simulink model "EPA_Jumper"  (R2018a)
settings: Solver=FixedStepDiscrete  StartTime=0.0  StopTime=inf  FixedStep=0.001  RelTol=1e-3  EnableMultiTasking=on
model workspace (MAT data in the model file):
  MCOS : class17 (value not decoded)
values from neighbouring files (symbols this model uses):
  bits_current = 12    [Init_EPA_Jumper.m]
  bits_Kd = 12    [Init_EPA_Jumper.m]
  bits_Kp = 12    [Init_EPA_Jumper.m]
  bits_position = 16    [Init_EPA_Jumper.m]
  bits_velocity = 12    [Init_EPA_Jumper.m]
  KD_MAX = 5.0    (= 5)    [Init_EPA_Jumper.m]
  KD_MIN = 0.0    (= 0)    [Init_EPA_Jumper.m]
  KP_MAX = 500.0    (= 500)    [Init_EPA_Jumper.m]
  KP_MIN = 0.0    (= 0)    [Init_EPA_Jumper.m]
  P_MAX = 95.5    [Init_EPA_Jumper.m]
  P_MIN = -95.5    [Init_EPA_Jumper.m]
  PressureFilter_CutOffFreq = 20    [Init_EPA_Jumper.m]
  PressureFilter_Gain = 1    [Init_EPA_Jumper.m]
  ReadingVoltage = 5    [Init_EPA_Jumper.m]
  T_MAX = 18.0    (= 18)    [Init_EPA_Jumper.m]
  T_MIN = -18.0    (= -18)    [Init_EPA_Jumper.m]
  V_MAX = 45.0    (= 45)    [Init_EPA_Jumper.m]
  V_MIN = -45.0    (= -45)    [Init_EPA_Jumper.m]
  voltageBias = -2.5    [Init_EPA_Jumper.m]
  voltageMultiplier = 2.5    [Init_EPA_Jumper.m]
  VoltageResolution = 1023.0    (= 1023)    [Init_EPA_Jumper.m]
libraries: xpcethercatlib x76, slrtlib x15, simulink x10, peGeneralControl x9
(part 2 of 3)

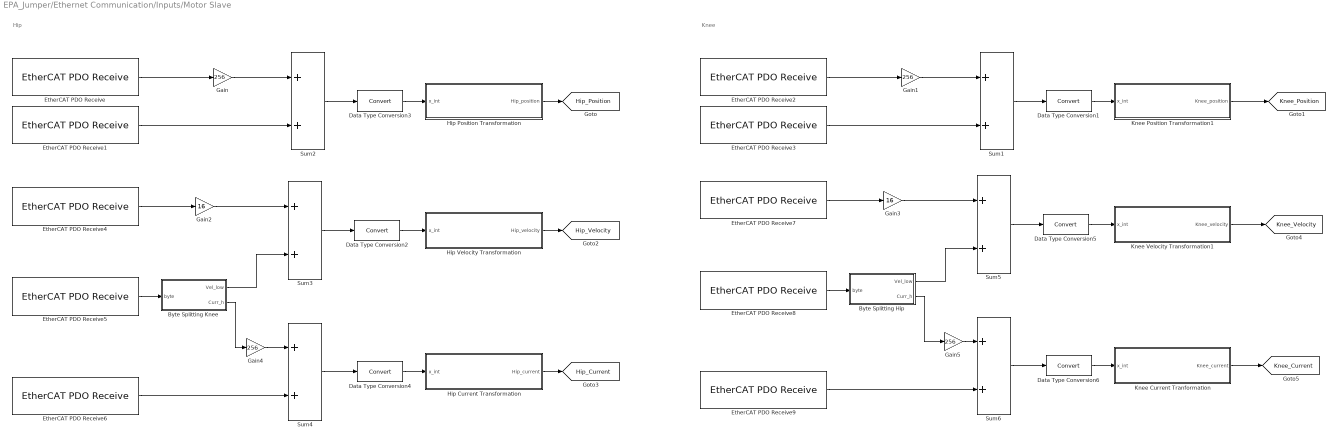
== system EPA_Jumper/Ethernet Communication/Inputs/Motor Slave ==
  note: Hip
  note: Knee
  Byte Splitting Hip : MATLAB Function  TreatAsAtomicUnit=on
  Byte Splitting Knee : MATLAB Function  TreatAsAtomicUnit=on
  Data Type Conversion{1..6} (6 alike) : DataTypeConversion
  EtherCAT PDO Receive : xpcethercatlib/EtherCAT PDO Receive  Priority=2  sig_name=Motors.Inputs.Byte0  sig_offset=464  sig_type=uint8  type_size=8  sig_dim=1  device_id=0  sample_time=0.001000
      settings: SourceProductName=Simulink Real-Time  SourceProductBaseCode=XP
  EtherCAT PDO Receive1 : xpcethercatlib/EtherCAT PDO Receive  Priority=2  sig_name=Motors.Inputs.Byte1  sig_offset=472  sig_type=uint8  type_size=8  sig_dim=1  device_id=0  sample_time=0.001000
      settings: SourceProductName=Simulink Real-Time  SourceProductBaseCode=XP
  EtherCAT PDO Receive2 : xpcethercatlib/EtherCAT PDO Receive  Priority=2  sig_name=Motors.Inputs.Byte5  sig_offset=504  sig_type=uint8  type_size=8  sig_dim=1  device_id=0  sample_time=0.001000
      settings: SourceProductName=Simulink Real-Time  SourceProductBaseCode=XP
  EtherCAT PDO Receive3 : xpcethercatlib/EtherCAT PDO Receive  Priority=2  sig_name=Motors.Inputs.Byte6  sig_offset=512  sig_type=uint8  type_size=8  sig_dim=1  device_id=0  sample_time=0.001000
      settings: SourceProductName=Simulink Real-Time  SourceProductBaseCode=XP
  EtherCAT PDO Receive4 : xpcethercatlib/EtherCAT PDO Receive  Priority=2  sig_name=Motors.Inputs.Byte2  sig_offset=480  sig_type=uint8  type_size=8  sig_dim=1  device_id=0  sample_time=0.001000
      settings: SourceProductName=Simulink Real-Time  SourceProductBaseCode=XP
  EtherCAT PDO Receive5 : xpcethercatlib/EtherCAT PDO Receive  Priority=2  sig_name=Motors.Inputs.Byte3  sig_offset=488  sig_type=uint8  type_size=8  sig_dim=1  device_id=0  sample_time=0.001000
      settings: SourceProductName=Simulink Real-Time  SourceProductBaseCode=XP
  EtherCAT PDO Receive6 : xpcethercatlib/EtherCAT PDO Receive  Priority=2  sig_name=Motors.Inputs.Byte4  sig_offset=496  sig_type=uint8  type_size=8  sig_dim=1  device_id=0  sample_time=0.001000
      settings: SourceProductName=Simulink Real-Time  SourceProductBaseCode=XP
  EtherCAT PDO Receive7 : xpcethercatlib/EtherCAT PDO Receive  Priority=2  sig_name=Motors.Inputs.Byte7  sig_offset=520  sig_type=uint8  type_size=8  sig_dim=1  device_id=0  sample_time=0.001000
      settings: SourceProductName=Simulink Real-Time  SourceProductBaseCode=XP
  EtherCAT PDO Receive8 : xpcethercatlib/EtherCAT PDO Receive  Priority=2  sig_name=Motors.Inputs.Byte8  sig_offset=528  sig_type=uint8  type_size=8  sig_dim=1  device_id=0  sample_time=0.001000
      settings: SourceProductName=Simulink Real-Time  SourceProductBaseCode=XP
  EtherCAT PDO Receive9 : xpcethercatlib/EtherCAT PDO Receive  Priority=2  sig_name=Motors.Inputs.Byte9  sig_offset=536  sig_type=uint8  type_size=8  sig_dim=1  device_id=0  sample_time=0.001000
      settings: SourceProductName=Simulink Real-Time  SourceProductBaseCode=XP
  Gain{,1,4..5} (4 alike) : Gain  Gain=256
  Gain2 : Gain  Gain=16
  Gain3 : Gain  Gain=16
  Hip Current Transformation : MATLAB Function  TreatAsAtomicUnit=on
  Hip Position Transformation : MATLAB Function  TreatAsAtomicUnit=on
  Hip Velocity Transformation : MATLAB Function  TreatAsAtomicUnit=on
  Knee Current Tranformation : MATLAB Function  TreatAsAtomicUnit=on
  Knee Position Transformation1 : MATLAB Function  TreatAsAtomicUnit=on
  Knee Velocity Transformation1 : MATLAB Function  TreatAsAtomicUnit=on
  Sum{1..6} (6 alike) : Sum
  tag scope: Hip_Current=global, Hip_Position=global, Hip_Velocity=global, Knee_Current=global, Knee_Position=global, Knee_Velocity=global
  wires:
  EtherCAT PDO Receive/1 -> Gain/1
  Sum2/1 -> Data Type Conversion3/1
  Data Type Conversion3/1 -> Hip Position Transformation/1(x_int)
  Gain/1 -> Sum2/1
  EtherCAT PDO Receive1/1 -> Sum2/2
  EtherCAT PDO Receive3/1 -> Sum1/2
  Gain1/1 -> Sum1/1
  Data Type Conversion1/1 -> Knee Position Transformation1/1(x_int)
  EtherCAT PDO Receive2/1 -> Gain1/1
  Sum1/1 -> Data Type Conversion1/1
  EtherCAT PDO Receive5/1 -> Byte Splitting Knee/1(byte)
  EtherCAT PDO Receive4/1 -> Gain2/1
  Gain2/1 -> Sum3/1
  Byte Splitting Knee/1(Vel_low) -> Sum3/2
  EtherCAT PDO Receive6/1 -> Sum4/2
  Data Type Conversion2/1 -> Hip Velocity Transformation/1(x_int)
  Sum3/1 -> Data Type Conversion2/1
  Data Type Conversion4/1 -> Hip Current Transformation/1(x_int)
  Sum4/1 -> Data Type Conversion4/1
  EtherCAT PDO Receive7/1 -> Gain3/1
  Sum5/1 -> Data Type Conversion5/1
  Gain3/1 -> Sum5/1
  EtherCAT PDO Receive9/1 -> Sum6/2
  EtherCAT PDO Receive8/1 -> Byte Splitting Hip/1(byte)
  Byte Splitting Hip/2(Curr_h) -> Gain5/1
  Sum6/1 -> Data Type Conversion6/1
  Byte Splitting Hip/1(Vel_low) -> Sum5/2
  Hip Position Transformation/1(Hip_position) -> [Hip_Position]
  Hip Velocity Transformation/1(Hip_velocity) -> [Hip_Velocity]
  Hip Current Transformation/1(Hip_current) -> [Hip_Current]
  Knee Position Transformation1/1(Knee_position) -> [Knee_Position]
  Knee Velocity Transformation1/1(Knee_velocity) -> [Knee_Velocity]
  Data Type Conversion5/1 -> Knee Velocity Transformation1/1(x_int)
  Knee Current Tranformation/1(Knee_current) -> [Knee_Current]
  Data Type Conversion6/1 -> Knee Current Tranformation/1(x_int)
  Gain4/1 -> Sum4/1
  Byte Splitting Knee/2(Curr_h) -> Gain4/1
  Gain5/1 -> Sum6/1

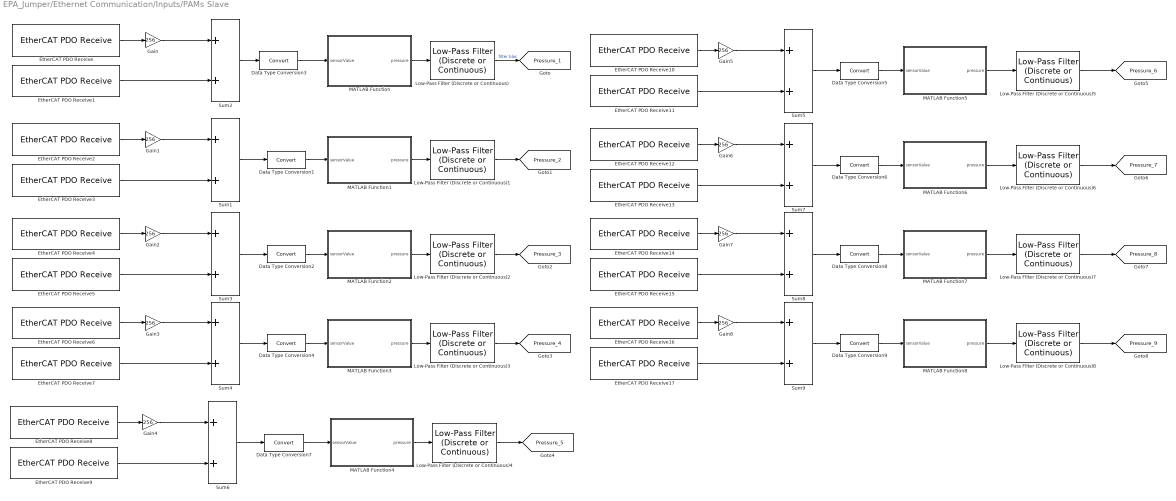
== system EPA_Jumper/Ethernet Communication/Inputs/PAMs Slave ==
  Data Type Conversion{1..9} (9 alike) : DataTypeConversion
  EtherCAT PDO Receive : xpcethercatlib/EtherCAT PDO Receive  Priority=2  sig_name=PAMs.Inputs.Byte0  sig_offset=720  sig_type=uint8  type_size=8  sig_dim=1  device_id=0  sample_time=0.001000
      settings: SourceProductName=Simulink Real-Time  SourceProductBaseCode=XP
  EtherCAT PDO Receive1 : xpcethercatlib/EtherCAT PDO Receive  Priority=2  sig_name=PAMs.Inputs.Byte1  sig_offset=728  sig_type=uint8  type_size=8  sig_dim=1  device_id=0  sample_time=0.001000
      settings: SourceProductName=Simulink Real-Time  SourceProductBaseCode=XP
  EtherCAT PDO Receive10 : xpcethercatlib/EtherCAT PDO Receive  Priority=2  sig_name=PAMs.Inputs.Byte10  sig_offset=800  sig_type=uint8  type_size=8  sig_dim=1  device_id=0  sample_time=0.001000
      settings: SourceProductName=Simulink Real-Time  SourceProductBaseCode=XP
  EtherCAT PDO Receive11 : xpcethercatlib/EtherCAT PDO Receive  Priority=2  sig_name=PAMs.Inputs.Byte11  sig_offset=808  sig_type=uint8  type_size=8  sig_dim=1  device_id=0  sample_time=0.001000
      settings: SourceProductName=Simulink Real-Time  SourceProductBaseCode=XP
  EtherCAT PDO Receive12 : xpcethercatlib/EtherCAT PDO Receive  Priority=2  sig_name=PAMs.Inputs.Byte12  sig_offset=816  sig_type=uint8  type_size=8  sig_dim=1  device_id=0  sample_time=0.001000
      settings: SourceProductName=Simulink Real-Time  SourceProductBaseCode=XP
  EtherCAT PDO Receive13 : xpcethercatlib/EtherCAT PDO Receive  Priority=2  sig_name=PAMs.Inputs.Byte13  sig_offset=824  sig_type=uint8  type_size=8  sig_dim=1  device_id=0  sample_time=0.001000
      settings: SourceProductName=Simulink Real-Time  SourceProductBaseCode=XP
  EtherCAT PDO Receive14 : xpcethercatlib/EtherCAT PDO Receive  Priority=2  sig_name=PAMs.Inputs.Byte14  sig_offset=832  sig_type=uint8  type_size=8  sig_dim=1  device_id=0  sample_time=0.001000
      settings: SourceProductName=Simulink Real-Time  SourceProductBaseCode=XP
  EtherCAT PDO Receive15 : xpcethercatlib/EtherCAT PDO Receive  Priority=2  sig_name=PAMs.Inputs.Byte15  sig_offset=840  sig_type=uint8  type_size=8  sig_dim=1  device_id=0  sample_time=0.001000
      settings: SourceProductName=Simulink Real-Time  SourceProductBaseCode=XP
  EtherCAT PDO Receive16 : xpcethercatlib/EtherCAT PDO Receive  Priority=2  sig_name=PAMs.Inputs.Byte16  sig_offset=848  sig_type=uint8  type_size=8  sig_dim=1  device_id=0  sample_time=0.001000
      settings: SourceProductName=Simulink Real-Time  SourceProductBaseCode=XP
  EtherCAT PDO Receive17 : xpcethercatlib/EtherCAT PDO Receive  Priority=2  sig_name=PAMs.Inputs.Byte17  sig_offset=856  sig_type=uint8  type_size=8  sig_dim=1  device_id=0  sample_time=0.001000
      settings: SourceProductName=Simulink Real-Time  SourceProductBaseCode=XP
  EtherCAT PDO Receive2 : xpcethercatlib/EtherCAT PDO Receive  Priority=2  sig_name=PAMs.Inputs.Byte2  sig_offset=736  sig_type=uint8  type_size=8  sig_dim=1  device_id=0  sample_time=0.001000
      settings: SourceProductName=Simulink Real-Time  SourceProductBaseCode=XP
  EtherCAT PDO Receive3 : xpcethercatlib/EtherCAT PDO Receive  Priority=2  sig_name=PAMs.Inputs.Byte3  sig_offset=744  sig_type=uint8  type_size=8  sig_dim=1  device_id=0  sample_time=0.001000
      settings: SourceProductName=Simulink Real-Time  SourceProductBaseCode=XP
  EtherCAT PDO Receive4 : xpcethercatlib/EtherCAT PDO Receive  Priority=2  sig_name=PAMs.Inputs.Byte4  sig_offset=752  sig_type=uint8  type_size=8  sig_dim=1  device_id=0  sample_time=0.001000
      settings: SourceProductName=Simulink Real-Time  SourceProductBaseCode=XP
  EtherCAT PDO Receive5 : xpcethercatlib/EtherCAT PDO Receive  Priority=2  sig_name=PAMs.Inputs.Byte5  sig_offset=760  sig_type=uint8  type_size=8  sig_dim=1  device_id=0  sample_time=0.001000
      settings: SourceProductName=Simulink Real-Time  SourceProductBaseCode=XP
  EtherCAT PDO Receive6 : xpcethercatlib/EtherCAT PDO Receive  Priority=2  sig_name=PAMs.Inputs.Byte6  sig_offset=768  sig_type=uint8  type_size=8  sig_dim=1  device_id=0  sample_time=0.001000
      settings: SourceProductName=Simulink Real-Time  SourceProductBaseCode=XP
  EtherCAT PDO Receive7 : xpcethercatlib/EtherCAT PDO Receive  Priority=2  sig_name=PAMs.Inputs.Byte7  sig_offset=776  sig_type=uint8  type_size=8  sig_dim=1  device_id=0  sample_time=0.001000
      settings: SourceProductName=Simulink Real-Time  SourceProductBaseCode=XP
  EtherCAT PDO Receive8 : xpcethercatlib/EtherCAT PDO Receive  Priority=2  sig_name=PAMs.Inputs.Byte8  sig_offset=784  sig_type=uint8  type_size=8  sig_dim=1  device_id=0  sample_time=0.001000
      settings: SourceProductName=Simulink Real-Time  SourceProductBaseCode=XP
  EtherCAT PDO Receive9 : xpcethercatlib/EtherCAT PDO Receive  Priority=2  sig_name=PAMs.Inputs.Byte9  sig_offset=792  sig_type=uint8  type_size=8  sig_dim=1  device_id=0  sample_time=0.001000
      settings: SourceProductName=Simulink Real-Time  SourceProductBaseCode=XP
  Gain{,1..8} (9 alike) : Gain  Gain=256
  Low-Pass Filter (Discrete or Continuous){,1..8} (9 alike) : peGeneralControl/Low-Pass Filter (Discrete or Continuous)  K=PressureFilter_Gain  T=1/PressureFilter_CutOffFreq  B=inf  A=-inf  Ts=-1
  MATLAB Function : MATLAB Function  TreatAsAtomicUnit=on
  MATLAB Function1 : MATLAB Function  TreatAsAtomicUnit=on
  MATLAB Function2 : MATLAB Function  TreatAsAtomicUnit=on
  MATLAB Function3 : MATLAB Function  TreatAsAtomicUnit=on
  MATLAB Function4 : MATLAB Function  TreatAsAtomicUnit=on
  MATLAB Function5 : MATLAB Function  TreatAsAtomicUnit=on
  MATLAB Function6 : MATLAB Function  TreatAsAtomicUnit=on
  MATLAB Function7 : MATLAB Function  TreatAsAtomicUnit=on
  MATLAB Function8 : MATLAB Function  TreatAsAtomicUnit=on
  Sum{1..9} (9 alike) : Sum
  tag scope: Pressure_1=global, Pressure_2=global, Pressure_3=global, Pressure_4=global, Pressure_5=global, Pressure_6=global, Pressure_7=global, Pressure_8=global, Pressure_9=global
  wires:
  EtherCAT PDO Receive1/1 -> Sum2/2
  Sum2/1 -> Data Type Conversion3/1
  EtherCAT PDO Receive/1 -> Gain/1
  Gain/1 -> Sum2/1
  Data Type Conversion3/1 -> MATLAB Function/1(sensorValue)
  Gain1/1 -> Sum1/1
  EtherCAT PDO Receive3/1 -> Sum1/2
  EtherCAT PDO Receive2/1 -> Gain1/1
  Data Type Conversion1/1 -> MATLAB Function1/1(sensorValue)
  Sum1/1 -> Data Type Conversion1/1
  Data Type Conversion2/1 -> MATLAB Function2/1(sensorValue)
  EtherCAT PDO Receive4/1 -> Gain2/1
  Gain2/1 -> Sum3/1
  Sum3/1 -> Data Type Conversion2/1
  EtherCAT PDO Receive5/1 -> Sum3/2
  Sum4/1 -> Data Type Conversion4/1
  Data Type Conversion4/1 -> MATLAB Function3/1(sensorValue)
  EtherCAT PDO Receive6/1 -> Gain3/1
  Gain3/1 -> Sum4/1
  EtherCAT PDO Receive7/1 -> Sum4/2
  Gain4/1 -> Sum6/1
  Sum6/1 -> Data Type Conversion7/1
  EtherCAT PDO Receive8/1 -> Gain4/1
  Data Type Conversion5/1 -> MATLAB Function5/1(sensorValue)
  EtherCAT PDO Receive10/1 -> Gain5/1
  Gain5/1 -> Sum5/1
  EtherCAT PDO Receive11/1 -> Sum5/2
  Data Type Conversion7/1 -> MATLAB Function4/1(sensorValue)
  EtherCAT PDO Receive15/1 -> Sum8/2
  Gain7/1 -> Sum8/1
  EtherCAT PDO Receive14/1 -> Gain7/1
  Data Type Conversion8/1 -> MATLAB Function7/1(sensorValue)
  Sum7/1 -> Data Type Conversion6/1
  Data Type Conversion6/1 -> MATLAB Function6/1(sensorValue)
  EtherCAT PDO Receive12/1 -> Gain6/1
  Sum5/1 -> Data Type Conversion5/1
  Sum8/1 -> Data Type Conversion8/1
  EtherCAT PDO Receive9/1 -> Sum6/2
  Gain6/1 -> Sum7/1
  EtherCAT PDO Receive13/1 -> Sum7/2
  MATLAB Function/1(pressure) -> Low-Pass Filter (Discrete or Continuous)/1
  MATLAB Function1/1(pressure) -> Low-Pass Filter (Discrete or Continuous)1/1
  MATLAB Function2/1(pressure) -> Low-Pass Filter (Discrete or Continuous)2/1
  MATLAB Function3/1(pressure) -> Low-Pass Filter (Discrete or Continuous)3/1
  MATLAB Function4/1(pressure) -> Low-Pass Filter (Discrete or Continuous)4/1
  MATLAB Function5/1(pressure) -> Low-Pass Filter (Discrete or Continuous)5/1
  MATLAB Function6/1(pressure) -> Low-Pass Filter (Discrete or Continuous)6/1
  MATLAB Function7/1(pressure) -> Low-Pass Filter (Discrete or Continuous)7/1
  Sum9/1 -> Data Type Conversion9/1
  EtherCAT PDO Receive16/1 -> Gain8/1
  Data Type Conversion9/1 -> MATLAB Function8/1(sensorValue)
  Gain8/1 -> Sum9/1
  MATLAB Function8/1(pressure) -> Low-Pass Filter (Discrete or Continuous)8/1
  EtherCAT PDO Receive17/1 -> Sum9/2
  Low-Pass Filter (Discrete or Continuous)/1 -> [Pressure_1]  "filter bloc"
  Low-Pass Filter (Discrete or Continuous)1/1 -> [Pressure_2]
  Low-Pass Filter (Discrete or Continuous)2/1 -> [Pressure_3]
  Low-Pass Filter (Discrete or Continuous)3/1 -> [Pressure_4]
  Low-Pass Filter (Discrete or Continuous)4/1 -> [Pressure_5]
  Low-Pass Filter (Discrete or Continuous)5/1 -> [Pressure_6]
  Low-Pass Filter (Discrete or Continuous)6/1 -> [Pressure_7]
  Low-Pass Filter (Discrete or Continuous)7/1 -> [Pressure_8]
  Low-Pass Filter (Discrete or Continuous)8/1 -> [Pressure_9]

== system EPA_Jumper/Ethernet Communication/Outputs/GRF Slave ==
  Data Type Conversion13 : DataTypeConversion
  EtherCAT PDO Transmit 2 : xpcethercatlib/EtherCAT PDO Transmit   Priority=3  sig_name=GRF.Outputs.Byte0  sig_offset=208  sig_type=uint8  type_size=8  sig_dim=1  device_id=0  sample_time=0.001000
      settings: SourceProductName=Simulink Real-Time  SourceProductBaseCode=XP
  wires:
  Data Type Conversion13/1 -> EtherCAT PDO Transmit 2/1
  [GRF_Operation_Mode] -> Data Type Conversion13/1

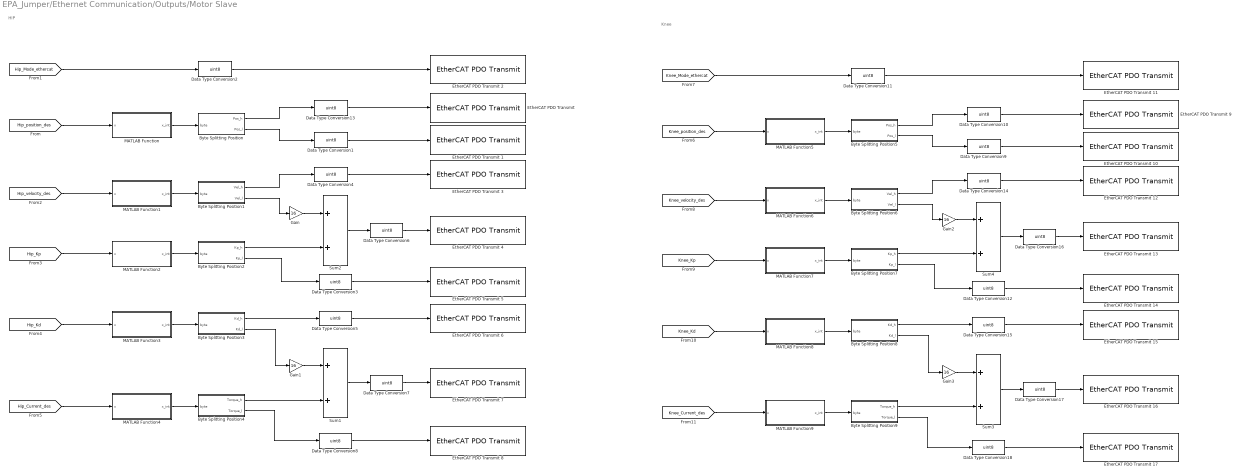
== system EPA_Jumper/Ethernet Communication/Outputs/Motor Slave ==
  note: HIP
  note: Knee
  Byte Splitting Position : MATLAB Function  TreatAsAtomicUnit=on
  Byte Splitting Position1 : MATLAB Function  TreatAsAtomicUnit=on
  Byte Splitting Position2 : MATLAB Function  TreatAsAtomicUnit=on
  Byte Splitting Position3 : MATLAB Function  TreatAsAtomicUnit=on
  Byte Splitting Position4 : MATLAB Function  TreatAsAtomicUnit=on
  Byte Splitting Position5 : MATLAB Function  TreatAsAtomicUnit=on
  Byte Splitting Position6 : MATLAB Function  TreatAsAtomicUnit=on
  Byte Splitting Position7 : MATLAB Function  TreatAsAtomicUnit=on
  Byte Splitting Position8 : MATLAB Function  TreatAsAtomicUnit=on
  Byte Splitting Position9 : MATLAB Function  TreatAsAtomicUnit=on
  Data Type Conversion{1,3..18} (17 alike) : DataTypeConversion  OutDataTypeStr=uint8
  Data Type Conversion2 : DataTypeConversion  OutDataTypeStr=uint8  RndMeth=Ceiling
  "EtherCAT PDO Transmit " : xpcethercatlib/EtherCAT PDO Transmit   Priority=3  sig_name=Motors.Outputs.Byte1  sig_offset=472  sig_type=uint8  type_size=8  sig_dim=1  device_id=0  sample_time=0.001000
      settings: SourceProductName=Simulink Real-Time  SourceProductBaseCode=XP
  EtherCAT PDO Transmit 1 : xpcethercatlib/EtherCAT PDO Transmit   Priority=3  sig_name=Motors.Outputs.Byte2  sig_offset=480  sig_type=uint8  type_size=8  sig_dim=1  device_id=0  sample_time=0.001000
      settings: SourceProductName=Simulink Real-Time  SourceProductBaseCode=XP
  EtherCAT PDO Transmit 10 : xpcethercatlib/EtherCAT PDO Transmit   Priority=3  sig_name=Motors.Outputs.Byte11  sig_offset=552  sig_type=uint8  type_size=8  sig_dim=1  device_id=0  sample_time=0.001000
      settings: SourceProductName=Simulink Real-Time  SourceProductBaseCode=XP
  EtherCAT PDO Transmit 11 : xpcethercatlib/EtherCAT PDO Transmit   Priority=3  sig_name=Motors.Outputs.Byte9  sig_offset=536  sig_type=uint8  type_size=8  sig_dim=1  device_id=0  sample_time=0.001000
      settings: SourceProductName=Simulink Real-Time  SourceProductBaseCode=XP
  EtherCAT PDO Transmit 12 : xpcethercatlib/EtherCAT PDO Transmit   Priority=3  sig_name=Motors.Outputs.Byte12  sig_offset=560  sig_type=uint8  type_size=8  sig_dim=1  device_id=0  sample_time=0.001000
      settings: SourceProductName=Simulink Real-Time  SourceProductBaseCode=XP
  EtherCAT PDO Transmit 13 : xpcethercatlib/EtherCAT PDO Transmit   Priority=3  sig_name=Motors.Outputs.Byte13  sig_offset=568  sig_type=uint8  type_size=8  sig_dim=1  device_id=0  sample_time=0.001000
      settings: SourceProductName=Simulink Real-Time  SourceProductBaseCode=XP
  EtherCAT PDO Transmit 14 : xpcethercatlib/EtherCAT PDO Transmit   Priority=3  sig_name=Motors.Outputs.Byte14  sig_offset=576  sig_type=uint8  type_size=8  sig_dim=1  device_id=0  sample_time=0.001000
      settings: SourceProductName=Simulink Real-Time  SourceProductBaseCode=XP
  EtherCAT PDO Transmit 15 : xpcethercatlib/EtherCAT PDO Transmit   Priority=3  sig_name=Motors.Outputs.Byte15  sig_offset=584  sig_type=uint8  type_size=8  sig_dim=1  device_id=0  sample_time=0.001000
      settings: SourceProductName=Simulink Real-Time  SourceProductBaseCode=XP
  EtherCAT PDO Transmit 16 : xpcethercatlib/EtherCAT PDO Transmit   Priority=3  sig_name=Motors.Outputs.Byte16  sig_offset=592  sig_type=uint8  type_size=8  sig_dim=1  device_id=0  sample_time=0.001000
      settings: SourceProductName=Simulink Real-Time  SourceProductBaseCode=XP
  EtherCAT PDO Transmit 17 : xpcethercatlib/EtherCAT PDO Transmit   Priority=3  sig_name=Motors.Outputs.Byte17  sig_offset=600  sig_type=uint8  type_size=8  sig_dim=1  device_id=0  sample_time=0.001000
      settings: SourceProductName=Simulink Real-Time  SourceProductBaseCode=XP
  EtherCAT PDO Transmit 2 : xpcethercatlib/EtherCAT PDO Transmit   Priority=3  sig_name=Motors.Outputs.Byte0  sig_offset=464  sig_type=uint8  type_size=8  sig_dim=1  device_id=0  sample_time=0.001000
      settings: SourceProductName=Simulink Real-Time  SourceProductBaseCode=XP
  EtherCAT PDO Transmit 3 : xpcethercatlib/EtherCAT PDO Transmit   Priority=3  sig_name=Motors.Outputs.Byte3  sig_offset=488  sig_type=uint8  type_size=8  sig_dim=1  device_id=0  sample_time=0.001000
      settings: SourceProductName=Simulink Real-Time  SourceProductBaseCode=XP
  EtherCAT PDO Transmit 4 : xpcethercatlib/EtherCAT PDO Transmit   Priority=3  sig_name=Motors.Outputs.Byte4  sig_offset=496  sig_type=uint8  type_size=8  sig_dim=1  device_id=0  sample_time=0.001000
      settings: SourceProductName=Simulink Real-Time  SourceProductBaseCode=XP
  EtherCAT PDO Transmit 5 : xpcethercatlib/EtherCAT PDO Transmit   Priority=3  sig_name=Motors.Outputs.Byte5  sig_offset=504  sig_type=uint8  type_size=8  sig_dim=1  device_id=0  sample_time=0.001000
      settings: SourceProductName=Simulink Real-Time  SourceProductBaseCode=XP
  EtherCAT PDO Transmit 6 : xpcethercatlib/EtherCAT PDO Transmit   Priority=3  sig_name=Motors.Outputs.Byte6  sig_offset=512  sig_type=uint8  type_size=8  sig_dim=1  device_id=0  sample_time=0.001000
      settings: SourceProductName=Simulink Real-Time  SourceProductBaseCode=XP
  EtherCAT PDO Transmit 7 : xpcethercatlib/EtherCAT PDO Transmit   Priority=3  sig_name=Motors.Outputs.Byte7  sig_offset=520  sig_type=uint8  type_size=8  sig_dim=1  device_id=0  sample_time=0.001000
      settings: SourceProductName=Simulink Real-Time  SourceProductBaseCode=XP
  EtherCAT PDO Transmit 8 : xpcethercatlib/EtherCAT PDO Transmit   Priority=3  sig_name=Motors.Outputs.Byte8  sig_offset=528  sig_type=uint8  type_size=8  sig_dim=1  device_id=0  sample_time=0.001000
      settings: SourceProductName=Simulink Real-Time  SourceProductBaseCode=XP
  EtherCAT PDO Transmit 9 : xpcethercatlib/EtherCAT PDO Transmit   Priority=3  sig_name=Motors.Outputs.Byte10  sig_offset=544  sig_type=uint8  type_size=8  sig_dim=1  device_id=0  sample_time=0.001000
      settings: SourceProductName=Simulink Real-Time  SourceProductBaseCode=XP
  Gain{,1..3} (4 alike) : Gain  Gain=16
  MATLAB Function : MATLAB Function  TreatAsAtomicUnit=on
  MATLAB Function1 : MATLAB Function  TreatAsAtomicUnit=on
  MATLAB Function2 : MATLAB Function  TreatAsAtomicUnit=on
  MATLAB Function3 : MATLAB Function  TreatAsAtomicUnit=on
  MATLAB Function4 : MATLAB Function  TreatAsAtomicUnit=on
  MATLAB Function5 : MATLAB Function  TreatAsAtomicUnit=on
  MATLAB Function6 : MATLAB Function  TreatAsAtomicUnit=on
  MATLAB Function7 : MATLAB Function  TreatAsAtomicUnit=on
  MATLAB Function8 : MATLAB Function  TreatAsAtomicUnit=on
  MATLAB Function9 : MATLAB Function  TreatAsAtomicUnit=on
  Sum{1..4} (4 alike) : Sum
  wires:
  [Hip_position_des] -> MATLAB Function/1(x)
  MATLAB Function/1(x_int) -> Byte Splitting Position/1(byte)
  Byte Splitting Position/1(Pos_h) -> Data Type Conversion13/1
  Byte Splitting Position/2(Pos_l) -> Data Type Conversion1/1
  Data Type Conversion13/1 -> "EtherCAT PDO Transmit "/1
  Data Type Conversion1/1 -> EtherCAT PDO Transmit 1/1
  [Hip_Mode_ethercat] -> Data Type Conversion2/1
  Data Type Conversion2/1 -> EtherCAT PDO Transmit 2/1
  MATLAB Function1/1(x_int) -> Byte Splitting Position1/1(byte)
  Byte Splitting Position1/1(Vel_h) -> Data Type Conversion4/1
  Byte Splitting Position1/2(Vel_l) -> Gain/1
  [Hip_velocity_des] -> MATLAB Function1/1(x)
  Data Type Conversion4/1 -> EtherCAT PDO Transmit 3/1
  Gain/1 -> Sum2/1
  Sum2/1 -> Data Type Conversion6/1
  [Hip_Kp] -> MATLAB Function2/1(x)
  MATLAB Function2/1(x_int) -> Byte Splitting Position2/1(byte)
  Byte Splitting Position2/1(Kp_h) -> Sum2/2
  Data Type Conversion3/1 -> EtherCAT PDO Transmit 5/1
  Byte Splitting Position2/2(Kp_l) -> Data Type Conversion3/1
  [Hip_Kd] -> MATLAB Function3/1(x)
  MATLAB Function3/1(x_int) -> Byte Splitting Position3/1(byte)
  Byte Splitting Position3/2(Kd_l) -> Gain1/1
  Byte Splitting Position3/1(Kd_h) -> Data Type Conversion5/1
  Sum1/1 -> Data Type Conversion7/1
  Data Type Conversion5/1 -> EtherCAT PDO Transmit 6/1
  Gain1/1 -> Sum1/1
  Data Type Conversion6/1 -> EtherCAT PDO Transmit 4/1
  Data Type Conversion7/1 -> EtherCAT PDO Transmit 7/1
  [Hip_Current_des] -> MATLAB Function4/1(x)
  MATLAB Function4/1(x_int) -> Byte Splitting Position4/1(byte)
  Byte Splitting Position4/2(Torque_l) -> Data Type Conversion8/1
  Byte Splitting Position4/1(Torque_h) -> Sum1/2
  Data Type Conversion8/1 -> EtherCAT PDO Transmit 8/1
  Byte Splitting Position9/2(Torque_l) -> Data Type Conversion18/1
  Data Type Conversion15/1 -> EtherCAT PDO Transmit 15/1
  Byte Splitting Position8/2(Kd_l) -> Gain3/1
  Data Type Conversion17/1 -> EtherCAT PDO Transmit 16/1
  MATLAB Function5/1(x_int) -> Byte Splitting Position5/1(byte)
  Data Type Conversion10/1 -> EtherCAT PDO Transmit 9/1
  Data Type Conversion18/1 -> EtherCAT PDO Transmit 17/1
  MATLAB Function9/1(x_int) -> Byte Splitting Position9/1(byte)
  Byte Splitting Position9/1(Torque_h) -> Sum3/2
  [Knee_Mode_ethercat] -> Data Type Conversion11/1
  Data Type Conversion14/1 -> EtherCAT PDO Transmit 12/1
  [Knee_Kp] -> MATLAB Function7/1(x)
  MATLAB Function7/1(x_int) -> Byte Splitting Position7/1(byte)
  Byte Splitting Position7/2(Kp_l) -> Data Type Conversion12/1
  Byte Splitting Position8/1(Kd_h) -> Data Type Conversion15/1
  [Knee_Current_des] -> MATLAB Function9/1(x)
  Byte Splitting Position6/2(Vel_l) -> Gain2/1
  Data Type Conversion12/1 -> EtherCAT PDO Transmit 14/1
  Sum3/1 -> Data Type Conversion17/1
  Byte Splitting Position7/1(Kp_h) -> Sum4/2
  Byte Splitting Position5/2(Pos_l) -> Data Type Conversion9/1
  Data Type Conversion9/1 -> EtherCAT PDO Transmit 10/1
  Byte Splitting Position5/1(Pos_h) -> Data Type Conversion10/1
  Sum4/1 -> Data Type Conversion16/1
  Data Type Conversion11/1 -> EtherCAT PDO Transmit 11/1
  [Knee_velocity_des] -> MATLAB Function6/1(x)
  [Knee_position_des] -> MATLAB Function5/1(x)
  [Knee_Kd] -> MATLAB Function8/1(x)
  Gain2/1 -> Sum4/1
  Gain3/1 -> Sum3/1
  MATLAB Function8/1(x_int) -> Byte Splitting Position8/1(byte)
  Byte Splitting Position6/1(Vel_h) -> Data Type Conversion14/1
  MATLAB Function6/1(x_int) -> Byte Splitting Position6/1(byte)
  Data Type Conversion16/1 -> EtherCAT PDO Transmit 13/1

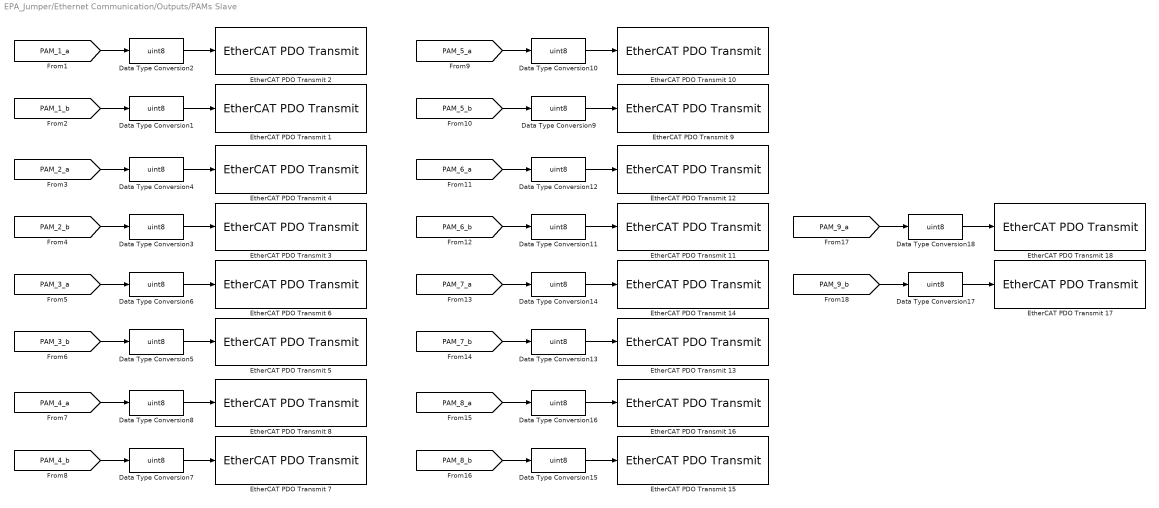
== system EPA_Jumper/Ethernet Communication/Outputs/PAMs Slave ==
  Data Type Conversion{1..18} (18 alike) : DataTypeConversion  OutDataTypeStr=uint8  RndMeth=Ceiling
  EtherCAT PDO Transmit 1 : xpcethercatlib/EtherCAT PDO Transmit   Priority=3  sig_name=PAMs.Outputs.Byte1  sig_offset=728  sig_type=uint8  type_size=8  sig_dim=1  device_id=0  sample_time=0.001000
      settings: SourceProductName=Simulink Real-Time  SourceProductBaseCode=XP
  EtherCAT PDO Transmit 10 : xpcethercatlib/EtherCAT PDO Transmit   Priority=3  sig_name=PAMs.Outputs.Byte8  sig_offset=784  sig_type=uint8  type_size=8  sig_dim=1  device_id=0  sample_time=0.001000
      settings: SourceProductName=Simulink Real-Time  SourceProductBaseCode=XP
  EtherCAT PDO Transmit 11 : xpcethercatlib/EtherCAT PDO Transmit   Priority=3  sig_name=PAMs.Outputs.Byte11  sig_offset=808  sig_type=uint8  type_size=8  sig_dim=1  device_id=0  sample_time=0.001000
      settings: SourceProductName=Simulink Real-Time  SourceProductBaseCode=XP
  EtherCAT PDO Transmit 12 : xpcethercatlib/EtherCAT PDO Transmit   Priority=3  sig_name=PAMs.Outputs.Byte10  sig_offset=800  sig_type=uint8  type_size=8  sig_dim=1  device_id=0  sample_time=0.001000
      settings: SourceProductName=Simulink Real-Time  SourceProductBaseCode=XP
  EtherCAT PDO Transmit 13 : xpcethercatlib/EtherCAT PDO Transmit   Priority=3  sig_name=PAMs.Outputs.Byte13  sig_offset=824  sig_type=uint8  type_size=8  sig_dim=1  device_id=0  sample_time=0.001000
      settings: SourceProductName=Simulink Real-Time  SourceProductBaseCode=XP
  EtherCAT PDO Transmit 14 : xpcethercatlib/EtherCAT PDO Transmit   Priority=3  sig_name=PAMs.Outputs.Byte12  sig_offset=816  sig_type=uint8  type_size=8  sig_dim=1  device_id=0  sample_time=0.001000
      settings: SourceProductName=Simulink Real-Time  SourceProductBaseCode=XP
  EtherCAT PDO Transmit 15 : xpcethercatlib/EtherCAT PDO Transmit   Priority=3  sig_name=PAMs.Outputs.Byte15  sig_offset=840  sig_type=uint8  type_size=8  sig_dim=1  device_id=0  sample_time=0.001000
      settings: SourceProductName=Simulink Real-Time  SourceProductBaseCode=XP
  EtherCAT PDO Transmit 16 : xpcethercatlib/EtherCAT PDO Transmit   Priority=3  sig_name=PAMs.Outputs.Byte14  sig_offset=832  sig_type=uint8  type_size=8  sig_dim=1  device_id=0  sample_time=0.001000
      settings: SourceProductName=Simulink Real-Time  SourceProductBaseCode=XP
  EtherCAT PDO Transmit 17 : xpcethercatlib/EtherCAT PDO Transmit   Priority=3  sig_name=PAMs.Outputs.Byte17  sig_offset=856  sig_type=uint8  type_size=8  sig_dim=1  device_id=0  sample_time=0.001000
      settings: SourceProductName=Simulink Real-Time  SourceProductBaseCode=XP
  EtherCAT PDO Transmit 18 : xpcethercatlib/EtherCAT PDO Transmit   Priority=3  sig_name=PAMs.Outputs.Byte16  sig_offset=848  sig_type=uint8  type_size=8  sig_dim=1  device_id=0  sample_time=0.001000
      settings: SourceProductName=Simulink Real-Time  SourceProductBaseCode=XP
  EtherCAT PDO Transmit 2 : xpcethercatlib/EtherCAT PDO Transmit   Priority=3  sig_name=PAMs.Outputs.Byte0  sig_offset=720  sig_type=uint8  type_size=8  sig_dim=1  device_id=0  sample_time=0.001000
      settings: SourceProductName=Simulink Real-Time  SourceProductBaseCode=XP
  EtherCAT PDO Transmit 3 : xpcethercatlib/EtherCAT PDO Transmit   Priority=3  sig_name=PAMs.Outputs.Byte3  sig_offset=744  sig_type=uint8  type_size=8  sig_dim=1  device_id=0  sample_time=0.001000
      settings: SourceProductName=Simulink Real-Time  SourceProductBaseCode=XP
  EtherCAT PDO Transmit 4 : xpcethercatlib/EtherCAT PDO Transmit   Priority=3  sig_name=PAMs.Outputs.Byte2  sig_offset=736  sig_type=uint8  type_size=8  sig_dim=1  device_id=0  sample_time=0.001000
      settings: SourceProductName=Simulink Real-Time  SourceProductBaseCode=XP
  EtherCAT PDO Transmit 5 : xpcethercatlib/EtherCAT PDO Transmit   Priority=3  sig_name=PAMs.Outputs.Byte5  sig_offset=760  sig_type=uint8  type_size=8  sig_dim=1  device_id=0  sample_time=0.001000
      settings: SourceProductName=Simulink Real-Time  SourceProductBaseCode=XP
  EtherCAT PDO Transmit 6 : xpcethercatlib/EtherCAT PDO Transmit   Priority=3  sig_name=PAMs.Outputs.Byte4  sig_offset=752  sig_type=uint8  type_size=8  sig_dim=1  device_id=0  sample_time=0.001000
      settings: SourceProductName=Simulink Real-Time  SourceProductBaseCode=XP
  EtherCAT PDO Transmit 7 : xpcethercatlib/EtherCAT PDO Transmit   Priority=3  sig_name=PAMs.Outputs.Byte7  sig_offset=776  sig_type=uint8  type_size=8  sig_dim=1  device_id=0  sample_time=0.001000
      settings: SourceProductName=Simulink Real-Time  SourceProductBaseCode=XP
  EtherCAT PDO Transmit 8 : xpcethercatlib/EtherCAT PDO Transmit   Priority=3  sig_name=PAMs.Outputs.Byte6  sig_offset=768  sig_type=uint8  type_size=8  sig_dim=1  device_id=0  sample_time=0.001000
      settings: SourceProductName=Simulink Real-Time  SourceProductBaseCode=XP
  EtherCAT PDO Transmit 9 : xpcethercatlib/EtherCAT PDO Transmit   Priority=3  sig_name=PAMs.Outputs.Byte9  sig_offset=792  sig_type=uint8  type_size=8  sig_dim=1  device_id=0  sample_time=0.001000
      settings: SourceProductName=Simulink Real-Time  SourceProductBaseCode=XP
  wires:
  Data Type Conversion2/1 -> EtherCAT PDO Transmit 2/1
  [PAM_1_a] -> Data Type Conversion2/1
  [PAM_1_b] -> Data Type Conversion1/1
  Data Type Conversion1/1 -> EtherCAT PDO Transmit 1/1
  Data Type Conversion3/1 -> EtherCAT PDO Transmit 3/1
  [PAM_2_a] -> Data Type Conversion4/1
  [PAM_2_b] -> Data Type Conversion3/1
  Data Type Conversion4/1 -> EtherCAT PDO Transmit 4/1
  Data Type Conversion6/1 -> EtherCAT PDO Transmit 6/1
  Data Type Conversion8/1 -> EtherCAT PDO Transmit 8/1
  [PAM_4_b] -> Data Type Conversion7/1
  [PAM_3_a] -> Data Type Conversion6/1
  [PAM_3_b] -> Data Type Conversion5/1
  [PAM_4_a] -> Data Type Conversion8/1
  Data Type Conversion7/1 -> EtherCAT PDO Transmit 7/1
  Data Type Conversion5/1 -> EtherCAT PDO Transmit 5/1
  [PAM_8_a] -> Data Type Conversion16/1
  Data Type Conversion16/1 -> EtherCAT PDO Transmit 16/1
  Data Type Conversion13/1 -> EtherCAT PDO Transmit 13/1
  [PAM_7_b] -> Data Type Conversion13/1
  [PAM_8_b] -> Data Type Conversion15/1
  [PAM_7_a] -> Data Type Conversion14/1
  Data Type Conversion14/1 -> EtherCAT PDO Transmit 14/1
  Data Type Conversion10/1 -> EtherCAT PDO Transmit 10/1
  Data Type Conversion12/1 -> EtherCAT PDO Transmit 12/1
  [PAM_6_b] -> Data Type Conversion11/1
  [PAM_5_a] -> Data Type Conversion10/1
  Data Type Conversion15/1 -> EtherCAT PDO Transmit 15/1
  [PAM_5_b] -> Data Type Conversion9/1
  [PAM_6_a] -> Data Type Conversion12/1
  Data Type Conversion11/1 -> EtherCAT PDO Transmit 11/1
  Data Type Conversion9/1 -> EtherCAT PDO Transmit 9/1
  Data Type Conversion17/1 -> EtherCAT PDO Transmit 17/1
  [PAM_9_a] -> Data Type Conversion18/1
  [PAM_9_b] -> Data Type Conversion17/1
  Data Type Conversion18/1 -> EtherCAT PDO Transmit 18/1

== system EPA_Jumper/High Level Control/Stance phase/FMCK (Static) ==
  GRF_Z : Inport
  angKne : Inport  Port=2
  C_ : Inport  Port=3
  Phi_0 : Inport  Port=4
  Add1 : Sum  Inputs=+-
  Gain2 : Gain
  Gain3 : Gain  Gain=pi/180
  Multiply1 : Product
  Multiply2 : Product
  torMotKne : Outport  InitialOutput=0
  Phi0 : Outport  Port=2  InitialOutput=0
  C : Outport  Port=3  InitialOutput=0
  wires:
  Add1/1 -> Gain3/1
  GRF_Z/1 -> Multiply1/1
  Multiply1/1 -> Multiply2/2
  angKne/1 -> Add1/1
  Multiply2/1 -> Gain2/1
  Phi_0/1 -> Add1/2, Phi0/1
  C_/1 -> C/1, Multiply2/1
  Gain2/1 -> torMotKne/1
  Gain3/1 -> Multiply1/2

== system EPA_Jumper/Ethernet Communication/Inputs/GRF Slave/GRFx  ==

== system EPA_Jumper/Ethernet Communication/Inputs/GRF Slave/GRFy  ==

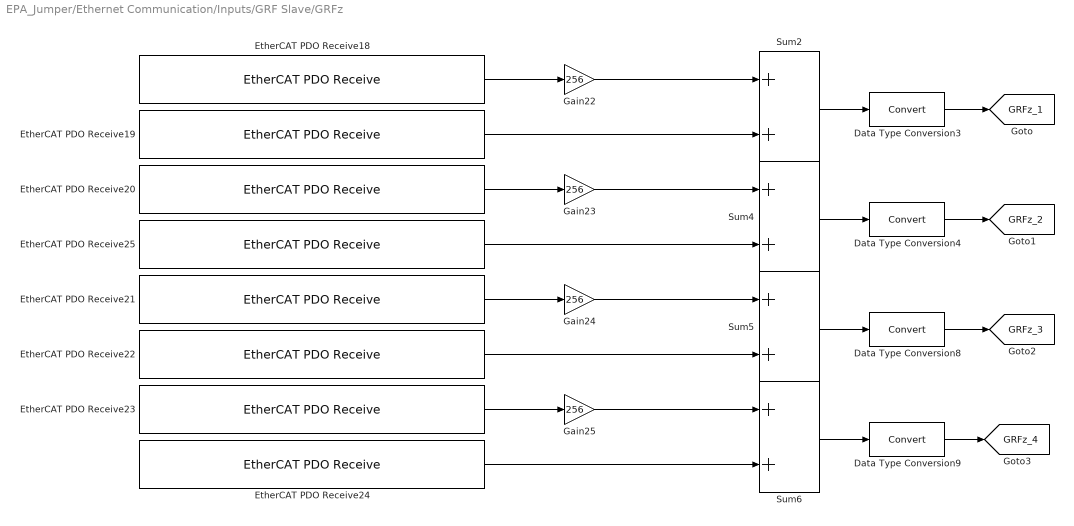
== system EPA_Jumper/Ethernet Communication/Inputs/GRF Slave/GRFz  ==
  Data Type Conversion{3..4,8..9} (4 alike) : DataTypeConversion
  EtherCAT PDO Receive18 : xpcethercatlib/EtherCAT PDO Receive  Priority=2  sig_name=GRF.Inputs.Byte0  sig_offset=208  sig_type=uint8  type_size=8  sig_dim=1  device_id=0  sample_time=0.001000
      settings: SourceProductName=Simulink Real-Time  SourceProductBaseCode=XP
  EtherCAT PDO Receive19 : xpcethercatlib/EtherCAT PDO Receive  Priority=2  sig_name=GRF.Inputs.Byte1  sig_offset=216  sig_type=uint8  type_size=8  sig_dim=1  device_id=0  sample_time=0.001000
      settings: SourceProductName=Simulink Real-Time  SourceProductBaseCode=XP
  EtherCAT PDO Receive20 : xpcethercatlib/EtherCAT PDO Receive  Priority=2  sig_name=GRF.Inputs.Byte2  sig_offset=224  sig_type=uint8  type_size=8  sig_dim=1  device_id=0  sample_time=0.001000
      settings: SourceProductName=Simulink Real-Time  SourceProductBaseCode=XP
  EtherCAT PDO Receive21 : xpcethercatlib/EtherCAT PDO Receive  Priority=2  sig_name=GRF.Inputs.Byte4  sig_offset=240  sig_type=uint8  type_size=8  sig_dim=1  device_id=0  sample_time=0.001000
      settings: SourceProductName=Simulink Real-Time  SourceProductBaseCode=XP
  EtherCAT PDO Receive22 : xpcethercatlib/EtherCAT PDO Receive  Priority=2  sig_name=GRF.Inputs.Byte5  sig_offset=248  sig_type=uint8  type_size=8  sig_dim=1  device_id=0  sample_time=0.001000
      settings: SourceProductName=Simulink Real-Time  SourceProductBaseCode=XP
  EtherCAT PDO Receive23 : xpcethercatlib/EtherCAT PDO Receive  Priority=2  sig_name=GRF.Inputs.Byte6  sig_offset=256  sig_type=uint8  type_size=8  sig_dim=1  device_id=0  sample_time=0.001000
      settings: SourceProductName=Simulink Real-Time  SourceProductBaseCode=XP
  EtherCAT PDO Receive24 : xpcethercatlib/EtherCAT PDO Receive  Priority=2  sig_name=GRF.Inputs.Byte7  sig_offset=264  sig_type=uint8  type_size=8  sig_dim=1  device_id=0  sample_time=0.001000
      settings: SourceProductName=Simulink Real-Time  SourceProductBaseCode=XP
  EtherCAT PDO Receive25 : xpcethercatlib/EtherCAT PDO Receive  Priority=2  sig_name=GRF.Inputs.Byte3  sig_offset=232  sig_type=uint8  type_size=8  sig_dim=1  device_id=0  sample_time=0.001000
      settings: SourceProductName=Simulink Real-Time  SourceProductBaseCode=XP
  Gain{22..25} (4 alike) : Gain  Gain=256
  Sum{2,4..6} (4 alike) : Sum
  tag scope: GRFz_1=global, GRFz_2=global, GRFz_3=global, GRFz_4=global
  wires:
  EtherCAT PDO Receive25/1 -> Sum4/2
  Sum2/1 -> Data Type Conversion3/1
  Sum5/1 -> Data Type Conversion8/1
  Sum6/1 -> Data Type Conversion9/1
  EtherCAT PDO Receive24/1 -> Sum6/2
  EtherCAT PDO Receive23/1 -> Gain25/1
  EtherCAT PDO Receive18/1 -> Gain22/1
  EtherCAT PDO Receive19/1 -> Sum2/2
  Sum4/1 -> Data Type Conversion4/1
  Data Type Conversion8/1 -> [GRFz_3]
  EtherCAT PDO Receive21/1 -> Gain24/1
  Gain24/1 -> Sum5/1
  EtherCAT PDO Receive20/1 -> Gain23/1
  Gain23/1 -> Sum4/1
  EtherCAT PDO Receive22/1 -> Sum5/2
  Gain25/1 -> Sum6/1
  Data Type Conversion3/1 -> [GRFz_1]
  Data Type Conversion4/1 -> [GRFz_2]
  Data Type Conversion9/1 -> [GRFz_4]
  Gain22/1 -> Sum2/1

== matlab function EPA_Jumper/Ethernet Communication/Inputs/Motor Slave/Byte Splitting Knee ==
  data: byte input; Vel_low output; Curr_h output
function [Vel_low,Curr_h] = fcn(byte)

Vel_low = bitshift(byte,-4);
Curr_h = bitand(byte,15);

== matlab function EPA_Jumper/Safety /System On/Emergency Switch ==
  data: Emergency_switch input; y output
function y = fcn(Emergency_switch)

if Emergency_switch == 255
    y = 0;
else
    y = 1;
end

== matlab function EPA_Jumper/Ethernet Communication/Inputs/Motor Slave/Byte Splitting Hip ==
  data: byte input; Vel_low output; Curr_h output
function [Vel_low,Curr_h] = fcn(byte)

Vel_low = bitshift(byte,-4);
Curr_h = bitand(byte,15);

== matlab function EPA_Jumper/Ethernet Communication/Inputs/Motor Slave/Hip Position Transformation ==
  data: x_int input; Hip_position output; P_MIN parameter; P_MAX parameter; bits_position parameter
function Hip_position = uint_to_float(x_int, P_MIN, P_MAX, bits_position)
    Hip_position = uint_to_float(x_int, P_MIN, P_MAX, bits_position);
end

== matlab function EPA_Jumper/Ethernet Communication/Inputs/Motor Slave/Knee Position Transformation1 ==
  data: x_int input; Knee_position output; P_MIN parameter; P_MAX parameter; bits_position parameter
function Knee_position = uint_to_float(x_int, P_MIN, P_MAX, bits_position)
    Knee_position = uint_to_float(x_int, P_MIN, P_MAX, bits_position);
end

== matlab function EPA_Jumper/Ethernet Communication/Inputs/Motor Slave/Hip Velocity Transformation ==
  data: x_int input; Hip_velocity output; V_MIN parameter; V_MAX parameter; bits_velocity parameter
function Hip_velocity = uint_to_float(x_int, V_MIN, V_MAX, bits_velocity)
    % Converts an unsigned int to float, given range and number of bits %
    Hip_velocity = uint_to_float(x_int, V_MIN, V_MAX, bits_velocity);

end

== matlab function EPA_Jumper/Ethernet Communication/Inputs/Motor Slave/Hip Current Transformation ==
  data: x_int input; Hip_current output; T_MIN parameter; T_MAX parameter; bits_current parameter
function Hip_current = uint_to_float(x_int, T_MIN, T_MAX, bits_current)
    % Converts an unsigned int to float, given range and number of bits %
    Hip_current = uint_to_float(x_int, T_MIN, T_MAX, bits_current);
end

== matlab function EPA_Jumper/Ethernet Communication/Inputs/Motor Slave/Knee Velocity Transformation1 ==
  data: x_int input; Knee_velocity output; V_MIN parameter; V_MAX parameter; bits_velocity parameter
function Knee_velocity = uint_to_float(x_int, V_MIN, V_MAX, bits_velocity)
    Knee_velocity = uint_to_float(x_int, V_MIN, V_MAX, bits_velocity);
end

== matlab function EPA_Jumper/Ethernet Communication/Inputs/Motor Slave/Knee Current Tranformation ==
  data: x_int input; Knee_current output; T_MIN parameter; T_MAX parameter; bits_current parameter
function Knee_current = uint_to_float(x_int, T_MIN, T_MAX, bits_current)
    Knee_current = uint_to_float(x_int, T_MIN, T_MAX, bits_current);
end

== matlab function EPA_Jumper/Ethernet Communication/Outputs/Motor Slave/MATLAB Function ==
  data: x input; x_int output; P_MIN parameter; P_MAX parameter; bits_position parameter
function x_int = float_to_uint(x, P_MIN, P_MAX, bits_position)
    % Converts a float to an unsigned int, given range and number of bits_position %
    x_int = float_to_uint(x, P_MIN, P_MAX, bits_position);
end

== matlab function EPA_Jumper/Ethernet Communication/Outputs/Motor Slave/Byte Splitting Position ==
  data: byte input; Pos_h output; Pos_l output
function [Pos_h,Pos_l] = fcn(byte)

Pos_l = bitand(byte,255);
Pos_h = bitshift(byte,-8);

== matlab function EPA_Jumper/Ethernet Communication/Outputs/Motor Slave/Byte Splitting Position1 ==
  data: byte input; Vel_h output; Vel_l output
function [Vel_h,Vel_l] = fcn(byte)

Vel_l = bitand(byte,15);
Vel_h = bitshift(byte,-4);

== matlab function EPA_Jumper/Ethernet Communication/Outputs/Motor Slave/MATLAB Function1 ==
  data: x input; x_int output; V_MIN parameter; V_MAX parameter; bits_velocity parameter
function x_int = float_to_uint(x, V_MIN, V_MAX, bits_velocity)
    % Converts a float to an unsigned int, given range and number of bits_velocity %
    x_int = float_to_uint(x, V_MIN, V_MAX, bits_velocity);
end

== matlab function EPA_Jumper/Ethernet Communication/Outputs/Motor Slave/Byte Splitting Position2 ==
  data: byte input; Kp_h output; Kp_l output
 function [Kp_h,Kp_l] = fcn(byte)

Kp_l = bitand(byte,255);
Kp_h = bitshift(byte,-8);

== matlab function EPA_Jumper/Ethernet Communication/Outputs/Motor Slave/MATLAB Function2 ==
  data: x input; x_int output; KP_MIN parameter; KP_MAX parameter; bits_Kp parameter
function x_int = float_to_uint(x, KP_MIN, KP_MAX, bits_Kp)
    % Converts a float to an unsigned int, given range and number of bits_Kp %
    x_int = float_to_uint(x, KP_MIN, KP_MAX, bits_Kp);

end

== matlab function EPA_Jumper/Ethernet Communication/Outputs/Motor Slave/Byte Splitting Position3 ==
  data: byte input; Kd_h output; Kd_l output
function [Kd_h,Kd_l] = fcn(byte)

Kd_l = bitand(byte,15);
Kd_h = bitshift(byte,-4);

== matlab function EPA_Jumper/Ethernet Communication/Outputs/Motor Slave/MATLAB Function3 ==
  data: x input; x_int output; KD_MIN parameter; KD_MAX parameter; bits_Kd parameter
function x_int = float_to_uint(x, KD_MIN, KD_MAX, bits_Kd)
    % Converts a float to an unsigned int, given range and number of bits_Kd %
    x_int = float_to_uint(x, KD_MIN, KD_MAX, bits_Kd);

end

== matlab function EPA_Jumper/Ethernet Communication/Outputs/Motor Slave/Byte Splitting Position4 ==
  data: byte input; Torque_h output; Torque_l output
function [Torque_h,Torque_l] = fcn(byte)

Torque_l = bitand(byte,255);
Torque_h = bitshift(byte,-8);

== matlab function EPA_Jumper/Ethernet Communication/Outputs/Motor Slave/MATLAB Function4 ==
  data: x input; x_int output; T_MIN parameter; T_MAX parameter; bits_current parameter
function x_int = float_to_uint(x, T_MIN, T_MAX, bits_current)
    % Converts a float to an unsigned int, given range and number of bits_current %
    x_int = float_to_uint(x, T_MIN, T_MAX, bits_current);

end

== matlab function EPA_Jumper/Ethernet Communication/Outputs/Motor Slave/Byte Splitting Position5 ==
  data: byte input; Pos_h output; Pos_l output
function [Pos_h,Pos_l] = fcn(byte)

Pos_l = bitand(byte,255);
Pos_h = bitshift(byte,-8);

== matlab function EPA_Jumper/Ethernet Communication/Outputs/Motor Slave/Byte Splitting Position6 ==
  data: byte input; Vel_h output; Vel_l output
function [Vel_h,Vel_l] = fcn(byte)

Vel_l = bitand(byte,15);
Vel_h = bitshift(byte,-4);

== matlab function EPA_Jumper/Ethernet Communication/Outputs/Motor Slave/Byte Splitting Position7 ==
  data: byte input; Kp_h output; Kp_l output
function [Kp_h,Kp_l] = fcn(byte)

Kp_l = bitand(byte,255);
Kp_h = bitshift(byte,-8);

== matlab function EPA_Jumper/Ethernet Communication/Outputs/Motor Slave/Byte Splitting Position8 ==
  data: byte input; Kd_h output; Kd_l output
function [Kd_h,Kd_l] = fcn(byte)

Kd_l = bitand(byte,15);
Kd_h = bitshift(byte,-4);

== matlab function EPA_Jumper/Ethernet Communication/Outputs/Motor Slave/Byte Splitting Position9 ==
  data: byte input; Torque_h output; Torque_l output
function [Torque_h,Torque_l] = fcn(byte)

Torque_l = bitand(byte,255);
Torque_h = bitshift(byte,-8);

== matlab function EPA_Jumper/Ethernet Communication/Outputs/Motor Slave/MATLAB Function5 ==
  data: x input; x_int output; P_MIN parameter; P_MAX parameter; bits_position parameter
function x_int = float_to_uint(x, P_MIN, P_MAX, bits_position)
    % Converts a float to an unsigned int, given range and number of bits_position %
    x_int = float_to_uint(x, P_MIN, P_MAX, bits_position);
end

== matlab function EPA_Jumper/Ethernet Communication/Outputs/Motor Slave/MATLAB Function6 ==
  data: x input; x_int output; V_MIN parameter; V_MAX parameter; bits_velocity parameter
function x_int = float_to_uint(x, V_MIN, V_MAX, bits_velocity)
    % Converts a float to an unsigned int, given range and number of bits_velocity %
    x_int = float_to_uint(x, V_MIN, V_MAX, bits_velocity);

end

== matlab function EPA_Jumper/Ethernet Communication/Outputs/Motor Slave/MATLAB Function7 ==
  data: x input; x_int output; KP_MIN parameter; KP_MAX parameter; bits_Kp parameter
function x_int = float_to_uint(x, KP_MIN, KP_MAX, bits_Kp)
    % Converts a float to an unsigned int, given range and number of bits_Kp %
    x_int = float_to_uint(x, KP_MIN, KP_MAX, bits_Kp);
end

== matlab function EPA_Jumper/Ethernet Communication/Outputs/Motor Slave/MATLAB Function8 ==
  data: x input; x_int output; KD_MIN parameter; KD_MAX parameter; bits_Kd parameter
function x_int = float_to_uint(x, KD_MIN, KD_MAX, bits_Kd)
    % Converts a float to an unsigned int, given range and number of bits_Kd %
    x_int = float_to_uint(x, KD_MIN, KD_MAX, bits_Kd);
end

== matlab function EPA_Jumper/Ethernet Communication/Outputs/Motor Slave/MATLAB Function9 ==
  data: x input; x_int output; T_MIN parameter; T_MAX parameter; bits_current parameter
function x_int = float_to_uint(x, T_MIN, T_MAX, bits_current)
    % Converts a float to an unsigned int, given range and number of bits_current %
    x_int = float_to_uint(x, T_MIN, T_MAX, bits_current);
end

== matlab function EPA_Jumper/Motors/Motor Mode Handler ==
  data: Hip_Mode input; Hip_Mode_out output; Hip_position_des input; Hip_velocity_des input; Hip_Kp input; Hip_Kd input; Hip_Curret_des input; Hip_position_des_out output; Hip_velocity_des_out output; Hip_Kp_out output; Hip_Kd_out output; Hip_Curret_des_out output
function [Hip_Mode_out, Hip_position_des_out, Hip_velocity_des_out, Hip_Kp_out, Hip_Kd_out, Hip_Curret_des_out] = fcn(Hip_Mode, Hip_position_des, Hip_velocity_des, Hip_Kp, Hip_Kd, Hip_Curret_des)

[Hip_Mode_out, Hip_position_des_out, Hip_velocity_des_out, Hip_Kp_out, Hip_Kd_out, Hip_Curret_des_out] = Motor_handler(Hip_Mode, Hip_position_des, Hip_velocity_des, Hip_Kp, Hip_Kd, Hip_Curret_des);

end

== matlab function EPA_Jumper/High Level Control/Hopping Phase Detection ==
  data: GRFz input; isFlight output
function isFlight = fcn(GRFz)

if GRFz > 5
    isFlight = 0;
else
    isFlight = 1;
end

end

== matlab function EPA_Jumper/Motors/Motor Mode Handler1 ==
  data: Knee_Mode input; Knee_Mode_out output; Knee_position_des input; Knee_velocity_des input; Knee_Kp input; Knee_Kd input; Knee_Curret_des input; Knee_position_des_out output; Knee_velocity_des_out output; Knee_Kp_out output; Knee_Kd_out output; Knee_Curret_des_out output
function [Knee_Mode_out, Knee_position_des_out, Knee_velocity_des_out, Knee_Kp_out, Knee_Kd_out, Knee_Curret_des_out] = fcn(Knee_Mode, Knee_position_des, Knee_velocity_des, Knee_Kp, Knee_Kd, Knee_Curret_des)

[Knee_Mode_out, Knee_position_des_out, Knee_velocity_des_out, Knee_Kp_out, Knee_Kd_out, Knee_Curret_des_out] = Motor_handler(Knee_Mode, Knee_position_des, Knee_velocity_des, Knee_Kp, Knee_Kd, Knee_Curret_des);

end

== matlab function EPA_Jumper/Safety /MATLAB Function ==
  data: Hip_motor_safe output; Knee_motor_safe output; Motors_safe output; flag output; Hip_Position input; Knee_Position input; flag_1 input
function [Hip_motor_safe, Knee_motor_safe,Motors_safe,flag]= fcn(Hip_Position, Knee_Position, flag_1)

flag = flag_1;
if flag == 0
    if Hip_Position >= -50 && Hip_Position <70
        Hip_motor_safe = 1;
    else
        Hip_motor_safe = 0;   
        flag = 1;
    end
    if Knee_Position >= -9 && Knee_Position <110
        Knee_motor_safe = 1;
    else
        Knee_motor_safe = 0;  
        flag = 1;
    end
    Motors_safe = double(Hip_motor_safe & Knee_motor_safe);
else
    if Hip_Position >= -50 && Hip_Position <70
        Hip_motor_safe = 1;
    else
        Hip_motor_safe = 0;   
        flag = 1;
    end

    if Knee_Position >= -9 && Knee_Position <110
        Knee_motor_safe = 1;
    else
        Knee_motor_safe = 0;  
        flag = 1;
    end
    Motors_safe = 0;
end

end

== matlab function EPA_Jumper/High Level Control/MATLAB Function ==
  data: isFligth input; Hip_mode output; Knee_mode output
function [Hip_mode, Knee_mode] = fcn(isFligth)

if isFligth == 1
    Hip_mode = 1;
    Knee_mode = 1;
elseif isFligth == 0
    Hip_mode = 2;
    Knee_mode = 2;
else
    Hip_mode = 0;
    Knee_mode = 0;
end
end
